simulink model "CTRL_SPECCTRL_FB_STRAT1_REG_test"  (R2024b)
settings: Solver=VariableStepAuto  StartTime=0.0  StopTime=10.0  RelTol=1e-3
libraries: CTRL_SPECCTRL_FB_STRAT1_REG x1
settings Model: Creator=blatak  LastModifiedBy=blatak

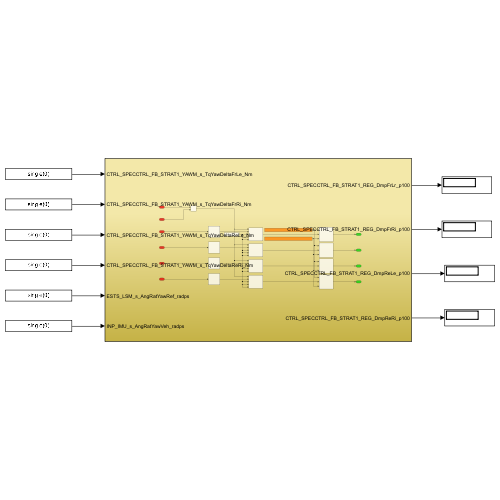
[thumbnail: Simulink's stored preview of the top-level diagram]
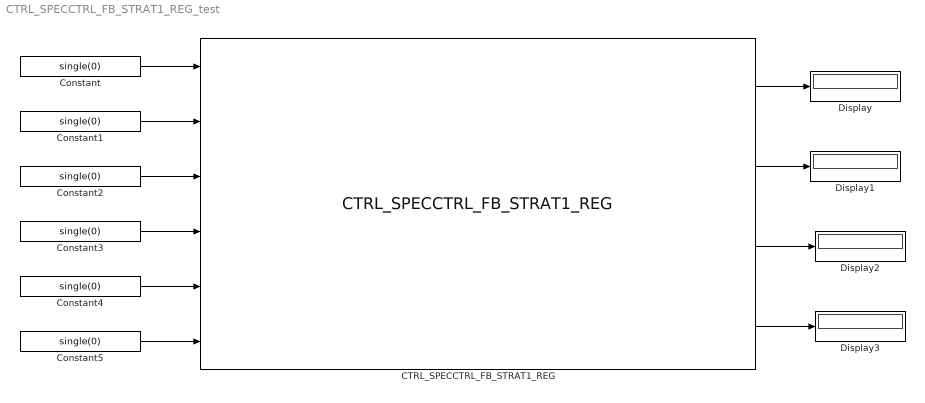
== system CTRL_SPECCTRL_FB_STRAT1_REG_test ==
  CTRL_SPECCTRL_FB_STRAT1_REG : CTRL_SPECCTRL_FB_STRAT1_REG/CTRL_SPECCTRL_FB_STRAT1_REG  SystemSampleTime=-1  VariantActivationTime=update diagram  AllowFlexibleInterface=on  Latency=0  AutoFrameSizeCalculation=off
  Constant{,1..5} (6 alike) : Constant  Value=single(0)
  Display{,1..3} (4 alike) : Display
  wires:
  Constant/1 -> CTRL_SPECCTRL_FB_STRAT1_REG/1
  Constant1/1 -> CTRL_SPECCTRL_FB_STRAT1_REG/2
  Constant2/1 -> CTRL_SPECCTRL_FB_STRAT1_REG/3
  Constant3/1 -> CTRL_SPECCTRL_FB_STRAT1_REG/4
  Constant4/1 -> CTRL_SPECCTRL_FB_STRAT1_REG/5
  Constant5/1 -> CTRL_SPECCTRL_FB_STRAT1_REG/6
  CTRL_SPECCTRL_FB_STRAT1_REG/1 -> Display/1
  CTRL_SPECCTRL_FB_STRAT1_REG/4 -> Display3/1
  CTRL_SPECCTRL_FB_STRAT1_REG/3 -> Display2/1
  CTRL_SPECCTRL_FB_STRAT1_REG/2 -> Display1/1
